simulink library "Yaw_Gearbox_Lib"  (Simulink 7.9)
settings: Solver=ode45  StartTime=0.0  StopTime=10.0  RelTol=1e-3
undefined symbols (not defined in the file): WT_Params
libraries: fl_lib x7, sdl_lib x4, nesl_utility x1
Description:
  | Copyright 2011 MathWorks, Inc.
settings Model: Creator=smiller  LastModifiedBy=smiller

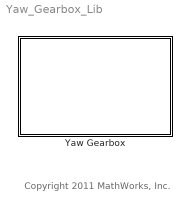
== system Yaw_Gearbox_Lib ==
  note: Copyright 2011 MathWorks, Inc.
  Yaw Gearbox : Subsystem
      mask Display: image(imread('Yaw_Gearbox_IMAGE.jpg'));

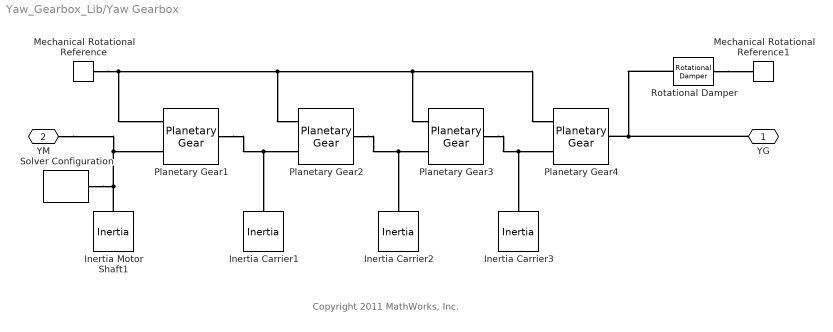
== system Yaw_Gearbox_Lib/Yaw Gearbox ==
  note: Copyright 2011 MathWorks, Inc.
  Inertia Carrier1 : fl_lib/Mechanical/Rotational Elements/Inertia  SystemSampleTime=-1  inertia=WT_Params.Yaw_Actuator.inertia_carrier kg*m^2  initial_velocity=0 rad/s  t_Log=off  LocalVarNames=|t  LocalVarDescs=|t  LocalVarLogging=0
  Inertia Carrier2 : fl_lib/Mechanical/Rotational Elements/Inertia  SystemSampleTime=-1  inertia=WT_Params.Yaw_Actuator.inertia_carrier kg*m^2  initial_velocity=0 rad/s  t_Log=off  LocalVarNames=|t  LocalVarDescs=|t  LocalVarLogging=0
  Inertia Carrier3 : fl_lib/Mechanical/Rotational Elements/Inertia  SystemSampleTime=-1  inertia=WT_Params.Yaw_Actuator.inertia_carrier kg*m^2  initial_velocity=0 rad/s  t_Log=off  LocalVarNames=|t  LocalVarDescs=|t  LocalVarLogging=0
  Inertia Motor Shaft1 : fl_lib/Mechanical/Rotational Elements/Inertia  inertia=WT_Params.Yaw_Actuator.inertia_motor_shaft kg*m^2  initial_velocity=0 rad/s  t_Log=off  LocalVarNames=|t  LocalVarDescs=|t  LocalVarLogging=0
  Mechanical Rotational Reference : fl_lib/Mechanical/Rotational Elements/Mechanical Rotational Reference  SystemSampleTime=-1  t_Log=off  LocalVarNames=|t  LocalVarDescs=|t  LocalVarLogging=0
  Mechanical Rotational Reference1 : fl_lib/Mechanical/Rotational Elements/Mechanical Rotational Reference  SystemSampleTime=-1  t_Log=off  LocalVarNames=|t  LocalVarDescs=|t  LocalVarLogging=0
  Planetary Gear1 : sdl_lib/Gears/Planetary Gear  rs_ratio=WT_Params.Yaw_Actuator.p_gear_rato_step_1-1  friction_model=1  efficiency=[ 0.96 0.98 ]  mu_visc=[ 0 0 ] N*m/(rad/s)  w_thr=[ 0.01 0.01 ] rad/s  LocalVarLogging=[]
  Planetary Gear2 : sdl_lib/Gears/Planetary Gear  SystemSampleTime=-1  rs_ratio=WT_Params.Yaw_Actuator.p_gear_rato_step_2-1  friction_model=1  efficiency=[ 0.96 0.98 ]  mu_visc=[ 0 0 ] N*m/(rad/s)  w_thr=[ 0.01 0.01 ] rad/s  LocalVarLogging=[]
  Planetary Gear3 : sdl_lib/Gears/Planetary Gear  SystemSampleTime=-1  rs_ratio=WT_Params.Yaw_Actuator.p_gear_rato_step_3-1  friction_model=1  efficiency=[ 0.96 0.98 ]  mu_visc=[ 0 0 ] N*m/(rad/s)  w_thr=[ 0.01 0.01 ] rad/s  LocalVarLogging=[]
  Planetary Gear4 : sdl_lib/Gears/Planetary Gear  rs_ratio=WT_Params.Yaw_Actuator.p_gear_rato_step_4-1  friction_model=1  efficiency=[ 0.96 0.98 ]  mu_visc=[ 0 0 ] N*m/(rad/s)  w_thr=[ 0.01 0.01 ] rad/s  LocalVarLogging=[]
  Rotational Damper : fl_lib/Mechanical/Rotational Elements/Rotational Damper  D=WT_Params.Yaw_Actuator.damping N*m/(rad/s)  t_Log=off  w_Log=off  LocalVarNames=|t|w  LocalVarDescs=|t|w  LocalVarLogging=[0 0]
  Solver Configuration : nesl_utility/Solver Configuration  PhysicalDomain=network_engine_domain  LeftPortType=input  RightPortType=generic  SubClassName=solver  UseCustomDae=off  DoDC=off  ResidualTolerance=1e-9  UseLocalSolver=off  LocalSolverChoice=NE_BACKWARD_EULER_ADVANCER  LocalSolverSampleTime=.001  DoFixedCost=off  MaxNonlinIter=12  MaxModeIter=2  LinearAlgebra=Sparse  Accelerate=off  Profile=off  UseLocalSampling=off  DelaysMemoryBudget=1024
  YG : PMIOPort  Port=1  Side=Right
  YM : PMIOPort  Port=2  Side=Left
  connections:
  Planetary Gear1/LConn1 -- Planetary Gear2/RConn2 -- Inertia Carrier1/LConn1
  Planetary Gear2/LConn1 -- Planetary Gear3/RConn2 -- Inertia Carrier2/LConn1
  Planetary Gear3/LConn1 -- Planetary Gear4/RConn2 -- Inertia Carrier3/LConn1
  Mechanical Rotational Reference/LConn1 -- Planetary Gear1/RConn1 -- Planetary Gear2/RConn1 -- Planetary Gear3/RConn1 -- Planetary Gear4/RConn1
  Inertia Motor Shaft1/LConn1 -- Planetary Gear1/RConn2 -- YM/RConn1 -- Solver Configuration/RConn1
  Rotational Damper/LConn1 -- YG/RConn1 -- Planetary Gear4/LConn1
  Rotational Damper/RConn1 -- Mechanical Rotational Reference1/LConn1
